simulink subsystem "Cell_elec_therm"  (R2019b)
settings: Solver=VariableStepAuto  StartTime=0.0  StopTime=10.0  RelTol=1e-3
values from neighbouring files (symbols this model uses):
  cell_prop = struct    [data_load.m]    (also in extend_model_ini.m = data_load('Cell_data.xlsx'))
libraries: fl_lib x10, nesl_utility x5, EpsaSimscape_lib x2
settings Model: Creator=ZHOU Jinhan  LastModifiedBy=ZHOU Jinhan

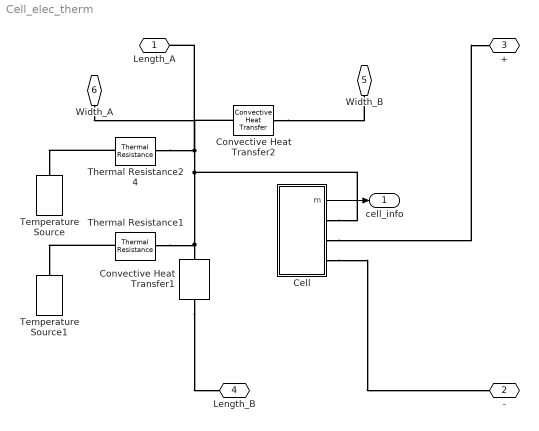
== system Cell_elec_therm ==
  Cell : Subsystem
  Convective Heat Transfer1 : fl_lib/Thermal/Thermal Elements/Convective Heat Transfer  area=cell_prop.cell_length*cell_prop.cell_height mm^2  heat_tr_coeff=10 W/(m^2 * K)  T_specify=off  T_priority=None  T=0 K  T_nominal_specify=off  T_nominal_unit=K  T_nominal_value=1  Q_specify=off  Q_priority=None  Q=0 W  Q_nominal_specify=off  Q_nominal_unit=W  Q_nominal_value=1
  Convective Heat Transfer2 : fl_lib/Thermal/Thermal Elements/Convective Heat Transfer  area=cell_prop.cell_width*cell_prop.cell_height mm^2  heat_tr_coeff=10 W/(m^2 * K)  T_specify=off  T_priority=None  T=0 K  T_nominal_specify=off  T_nominal_unit=K  T_nominal_value=1  Q_specify=off  Q_priority=None  Q=0 W  Q_nominal_specify=off  Q_nominal_unit=W  Q_nominal_value=1
  Temperature Source : fl_lib/Thermal/Thermal Sources/Temperature Source  temperature=cell_prop.T_ext K
      settings: SourceProductName=Simscape
  Temperature Source1 : fl_lib/Thermal/Thermal Sources/Temperature Source  temperature=cell_prop.T_ext K
      settings: SourceProductName=Simscape
  Thermal Resistance1 : fl_lib/Thermal/Thermal Elements/Thermal Resistance  resistance=1/cell_prop.cell_height*cell_prop.cell_length*cell_prop.wall*0.007874*0.4773 K/W  T_specify=off  T_priority=None  T=0 K  T_nominal_specify=off  T_nominal_unit=K  T_nominal_value=1  Q_specify=off  Q_priority=None  Q=0 W  Q_nominal_specify=off  Q_nominal_unit=W  Q_nominal_value=1
      settings: SourceProductName=Simscape  SourceProductBaseCode=SS
  Thermal Resistance24 : fl_lib/Thermal/Thermal Elements/Thermal Resistance  resistance=1/cell_prop.cell_height*cell_prop.cell_length*cell_prop.wall*0.007874*0.4773 K/W  T_specify=off  T_priority=None  T=0 K  T_nominal_specify=off  T_nominal_unit=K  T_nominal_value=1  Q_specify=off  Q_priority=None  Q=0 W  Q_nominal_specify=off  Q_nominal_unit=W  Q_nominal_value=1
      settings: SourceProductName=Simscape  SourceProductBaseCode=SS
  Length_A : PMIOPort  Side=Left
  - : PMIOPort  Port=2  Side=Right
  + : PMIOPort  Port=3  Side=Right
  Length_B : PMIOPort  Port=4  Side=Right
  Width_B : PMIOPort  Port=5  Side=Right
  Width_A : PMIOPort  Port=6  Side=Right
  cell_info : Outport
  wires:
  Cell/1(m) -> cell_info/1
  connections:
  Convective Heat Transfer1/LConn1 -- Cell/RConn1 -- Thermal Resistance24/LConn1 -- Width_A/RConn1 -- Convective Heat Transfer2/LConn1 -- Length_A/RConn1 -- Thermal Resistance1/LConn1
  Thermal Resistance1/RConn1 -- Temperature Source1/LConn1
  Thermal Resistance24/RConn1 -- Temperature Source/LConn1
  Convective Heat Transfer2/RConn1 -- Width_B/RConn1
  Cell/RConn2 -- +/RConn1
  Convective Heat Transfer1/RConn1 -- Length_B/RConn1
  Cell/RConn3 -- -/RConn1

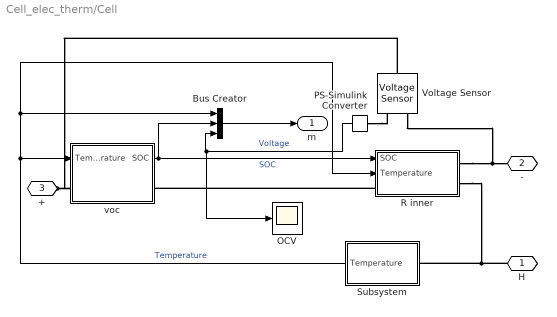
== system Cell_elec_therm/Cell ==
  Bus Creator : BusCreator  Inputs=3
  OCV : Scope
  PS-Simulink Converter : nesl_utility/PS-Simulink Converter  PhysicalDomain=network_engine_domain  SubClassName=ps_output  LeftPortType=input  RightPortType=output  PseudoPeriodic=off  Frequencies=[]  Unit=inherit  AffineConversion=off
  R inner : Subsystem
  Subsystem : Subsystem
  Voltage Sensor : fl_lib/Electrical/Electrical Sensors/Voltage Sensor
  voc : Subsystem
  H : PMIOPort  Side=Right
  - : PMIOPort  Port=2  Side=Right
  + : PMIOPort  Port=3  Side=Right
  m : Outport
  wires:
  Bus Creator/1 -> m/1
  voc/1(SOC) -> R inner/1(SOC), Bus Creator/2  "SOC"
  Subsystem/1(Temperature) -> R inner/2(Temperature), Bus Creator/1, voc/1(Temperature)  "Temperature"
  PS-Simulink Converter/1 -> OCV/1, Bus Creator/3  "Voltage"
  connections:
  voc/LConn1 -- +/RConn1 -- Voltage Sensor/LConn1
  Voltage Sensor/RConn2 -- -/RConn1 -- R inner/RConn1
  H/RConn1 -- R inner/RConn2 -- Subsystem/LConn1
  PS-Simulink Converter/LConn1 -- Voltage Sensor/RConn1
  R inner/LConn1 -- voc/RConn1

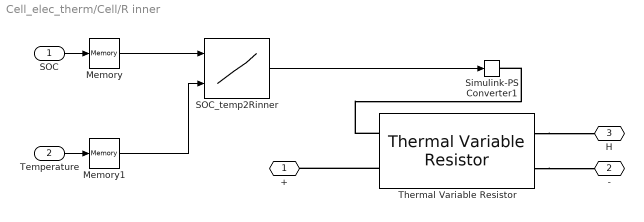
== system Cell_elec_therm/Cell/R inner ==
  SOC : Inport
  Temperature : Inport  Port=2
  Memory : Memory  InitialCondition=1  InheritSampleTime=on  LinearizeMemory=on
  Memory1 : Memory  InitialCondition=cell_prop.T_ext-273.15  InheritSampleTime=on  LinearizeMemory=on
  SOC_temp2Rinner : Lookup_n-D  BreakpointsForDimension1=cell_prop.R_in.SOC  BreakpointsForDimension2=cell_prop.R_in.T  Table=cell_prop.R_in.Rin/1000  ExtrapMethod=Clip  UseLastTableValue=on  InternalRulePriority=Speed  RndMeth=Simplest  InputSameDT=on
  Simulink-PS Converter1 : nesl_utility/Simulink-PS Converter  PhysicalDomain=network_engine_domain  SubClassName=ps_input  LeftPortType=input  RightPortType=output  PseudoPeriodic=off  Frequencies=[]  NoiseDistribution=none  NoiseParameters=[]  Unit=1  AffineConversion=off  FilteringAndDerivatives=provide  SimscapeFilterOrder=1  InputFilterTimeConstant=0.001  UdotUserProvided=0
  Thermal Variable Resistor : EpsaSimscape_lib/Thermal Variable Resistor  T0=273.15 K  tc=1 s  K_d=1.03*cell_prop.m_cell W/K  T_specify=off  T_priority=High  T=300 K  T_nominal_specify=off  T_nominal_unit=K  T_nominal_value=1
      settings: InternalSimscapePortConfiguration="{\"Bottom\":[],\"Left\":[{\"id\":\"R\",\"label\":\"R\",\"type\":\"input\"},{\"id\":\"p\",\"label\":\"+\",\"type\":\"foundation.electrical.electrical\"}],\"Right\":[{\"id\":\"H\",\"label\":\"H\",\"type\":\"foundation.thermal.thermal\"},{\"id\":\"n\",\"label\":\"-\",\"type\":\"foundation.electrical.electrical\"}],\"Top\":[]}"
  + : PMIOPort  Side=Left
  - : PMIOPort  Port=2  Side=Right
  H : PMIOPort  Port=3  Side=Right
  wires:
  SOC/1 -> Memory/1
  Temperature/1 -> Memory1/1
  SOC_temp2Rinner/1 -> Simulink-PS Converter1/1
  Memory/1 -> SOC_temp2Rinner/1
  Memory1/1 -> SOC_temp2Rinner/2
  connections:
  Thermal Variable Resistor/LConn2 -- +/RConn1
  Thermal Variable Resistor/LConn1 -- Simulink-PS Converter1/RConn1
  Thermal Variable Resistor/RConn2 -- -/RConn1
  Thermal Variable Resistor/RConn1 -- H/RConn1

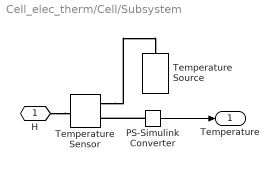
== system Cell_elec_therm/Cell/Subsystem ==
  PS-Simulink Converter : nesl_utility/PS-Simulink Converter  PhysicalDomain=network_engine_domain  SubClassName=ps_output  LeftPortType=input  RightPortType=output  PseudoPeriodic=off  Frequencies=[]  Unit=inherit  AffineConversion=off
  Temperature Sensor : fl_lib/Thermal/Thermal Sensors/Temperature Sensor
  Temperature Source : fl_lib/Thermal/Thermal Sources/Temperature Source  temperature=273.15 K
      settings: SourceProductName=Simscape
  H : PMIOPort  Side=Left
  Temperature : Outport
  wires:
  PS-Simulink Converter/1 -> Temperature/1
  connections:
  Temperature Sensor/RConn1 -- Temperature Source/LConn1
  H/RConn1 -- Temperature Sensor/LConn1
  PS-Simulink Converter/LConn1 -- Temperature Sensor/RConn2

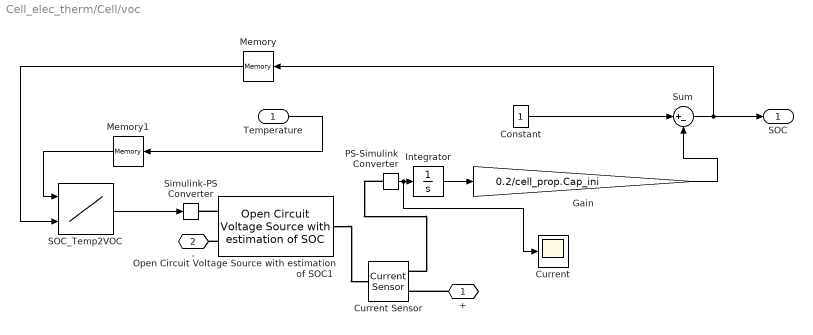
== system Cell_elec_therm/Cell/voc ==
  Temperature : Inport
  Constant : Constant
  Current : Scope
  Current Sensor : fl_lib/Electrical/Electrical Sensors/Current Sensor
  Gain : Gain  Gain=0.2/cell_prop.Cap_ini  ParamDataTypeStr=double
  Integrator : Integrator  LimitOutput=on  UpperSaturationLimit=1  LowerSaturationLimit=0
  Memory : Memory  InitialCondition=1  InheritSampleTime=on  LinearizeMemory=on
  Memory1 : Memory  InitialCondition=cell_prop.T_ext-273.15  InheritSampleTime=on  LinearizeMemory=on
  Open Circuit Voltage Source with estimation of SOC1 : EpsaSimscape_lib/Open Circuit Voltage Source with estimation of SOC  toVoltage=1 V
      settings: InternalSimscapePortConfiguration="{\"Bottom\":[],\"Left\":[{\"id\":\"p\",\"label\":\"+\",\"type\":\"foundation.electrical.electrical\"}],\"Right\":[{\"id\":\"OCV\",\"label\":\"OCV\",\"type\":\"input\"},{\"id\":\"n\",\"label\":\"-\",\"type\":\"foundation.electrical.electrical\"}],\"Top\":[]}"
  PS-Simulink Converter : nesl_utility/PS-Simulink Converter  PhysicalDomain=network_engine_domain  SubClassName=ps_output  LeftPortType=input  RightPortType=output  PseudoPeriodic=off  Frequencies=[]  Unit=inherit  AffineConversion=off
  "SOC_Temp2VOC " : Lookup_n-D  BreakpointsForDimension1=cell_prop.OCV.SOC  BreakpointsForDimension2=cell_prop.OCV.T  Table=cell_prop.OCV.ocv  ExtrapMethod=Clip  UseLastTableValue=on  InternalRulePriority=Speed  RndMeth=Simplest  InputSameDT=on
  Simulink-PS Converter : nesl_utility/Simulink-PS Converter  PhysicalDomain=network_engine_domain  SubClassName=ps_input  LeftPortType=input  RightPortType=output  PseudoPeriodic=off  Frequencies=[]  NoiseDistribution=none  NoiseParameters=[]  Unit=1  AffineConversion=off  FilteringAndDerivatives=provide  SimscapeFilterOrder=1  InputFilterTimeConstant=0.001  UdotUserProvided=0
  Sum : Sum  Inputs=|+-
  + : PMIOPort  Side=Left
  - : PMIOPort  Port=2  Side=Right
  SOC : Outport
  wires:
  Constant/1 -> Sum/1
  Gain/1 -> Sum/2
  Integrator/1 -> Gain/1
  "SOC_Temp2VOC "/1 -> Simulink-PS Converter/1
  Temperature/1 -> Memory1/1
  Sum/1 -> Memory/1, SOC/1
  Memory/1 -> "SOC_Temp2VOC "/2
  Memory1/1 -> "SOC_Temp2VOC "/1
  PS-Simulink Converter/1 -> Current/1, Integrator/1
  connections:
  +/RConn1 -- Current Sensor/RConn2
  PS-Simulink Converter/LConn1 -- Current Sensor/RConn1
  Open Circuit Voltage Source with estimation of SOC1/RConn1 -- Simulink-PS Converter/RConn1
  Open Circuit Voltage Source with estimation of SOC1/RConn2 -- -/RConn1
  Open Circuit Voltage Source with estimation of SOC1/LConn1 -- Current Sensor/LConn1
